simulink model "non_linear_model"  (Simulink 7.3)
settings: Solver=ode45  StartTime=0.0  StopTime=0.01  FixedStep=0.000001  RelTol=1e-1
libraries: simulink x3
settings Model: Creator=alex  LastModifiedBy=alex  BufferReuse=off
settings DataIOCC: SignalLoggingName=sigsOut
settings OptimizationCC: InlineInvariantSignals=on  OptimizeBlockIOStorage=off  BufferReuse=off  ExpressionFolding=off  LocalBlockOutputs=off
settings DebuggingCC: SaveWithParameterizedLinksMsg=none  SignalResolutionControl=TryResolveAllWithWarning  SolverPrmCheckMsg=none  MultiTaskDSMMsg=warning  MultiTaskCondExecSysMsg=none  StrictBusMsg=None
settings HardwareCC: TargetUnknown=on
settings RTWCC: IncludeERTFirstTime=on

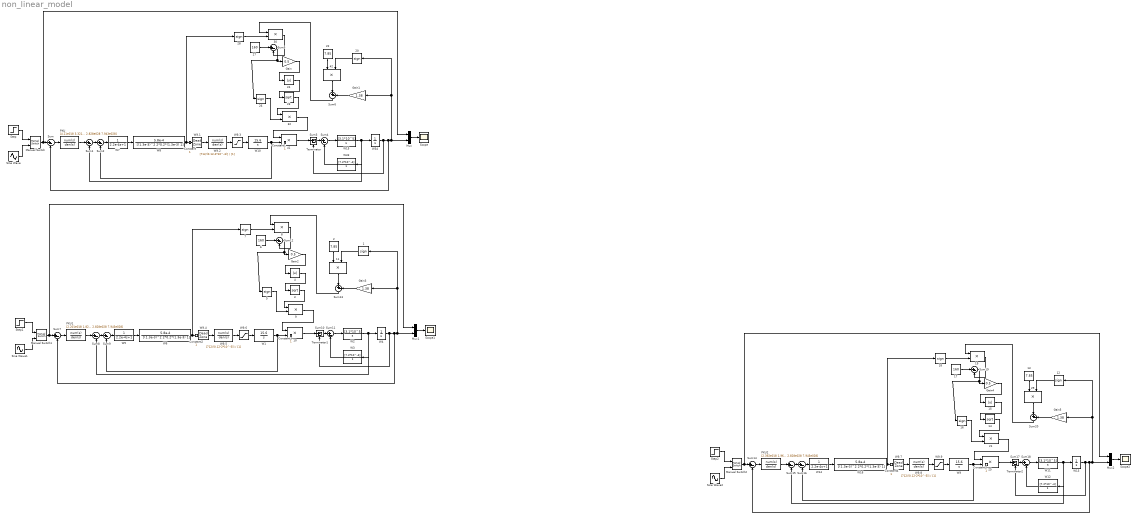
== system non_linear_model ==
  {1,5,7,12,16,18,20,26,28} (9 alike) : Signum
  {8..11,19,21,25,29..30,32,41..42} (12 alike) : Product  OutDataType=sfix(16)  OutScaling=2^0  SaturateOnIntegerOverflow=on  OutDataTypeStr=Inherit: Same as first input
  13 : Constant  Value=7.85  OutDataType=sfix(16)  OutScaling=2^0
  14 : Math  Operator=sqrt  SaturateOnIntegerOverflow=on
  15 : Abs  SaturateOnIntegerOverflow=on
  17 : Constant  Value=160  OutDataType=sfix(16)  OutScaling=2^0
  2 : Constant  Value=7.85  OutDataType=sfix(16)  OutScaling=2^0
  22 : Constant  Value=7.85  OutDataType=sfix(16)  OutScaling=2^0
  23 : Math  Operator=sqrt  SaturateOnIntegerOverflow=on
  24 : Abs  SaturateOnIntegerOverflow=on
  27 : Constant  Value=160  OutDataType=sfix(16)  OutScaling=2^0
  3 : Math  Operator=sqrt  SaturateOnIntegerOverflow=on
  4 : Abs  SaturateOnIntegerOverflow=on
  6 : Constant  Value=160  OutDataType=sfix(16)  OutScaling=2^0
  Constant{,1..5} (6 alike) : Constant  OutDataType=sfix(16)  OutScaling=2^0
  Gain : Gain  Gain=0.5  ParameterDataType=sfix(16)  ParameterScaling=2^0  OutDataType=sfix(16)  OutScaling=2^0  SaturateOnIntegerOverflow=on  OutDataTypeStr=Inherit: Same as input  ParamDataTypeStr=Inherit: Same as input
  Gain1 : Gain  Gain=1.38  ParameterDataType=sfix(16)  ParameterScaling=2^0  OutDataType=sfix(16)  OutScaling=2^0  SaturateOnIntegerOverflow=on  OutDataTypeStr=Inherit: Same as input  ParamDataTypeStr=Inherit: Same as input
  Gain2 : Gain  Gain=0.5  ParameterDataType=sfix(16)  ParameterScaling=2^0  OutDataType=sfix(16)  OutScaling=2^0  SaturateOnIntegerOverflow=on  OutDataTypeStr=Inherit: Same as input  ParamDataTypeStr=Inherit: Same as input
  Gain3 : Gain  Gain=1.38  ParameterDataType=sfix(16)  ParameterScaling=2^0  OutDataType=sfix(16)  OutScaling=2^0  SaturateOnIntegerOverflow=on  OutDataTypeStr=Inherit: Same as input  ParamDataTypeStr=Inherit: Same as input
  Gain4 : Gain  Gain=0.5  ParameterDataType=sfix(16)  ParameterScaling=2^0  OutDataType=sfix(16)  OutScaling=2^0  SaturateOnIntegerOverflow=on  OutDataTypeStr=Inherit: Same as input  ParamDataTypeStr=Inherit: Same as input
  Gain5 : Gain  Gain=1.38  ParameterDataType=sfix(16)  ParameterScaling=2^0  OutDataType=sfix(16)  OutScaling=2^0  SaturateOnIntegerOverflow=on  OutDataTypeStr=Inherit: Same as input  ParamDataTypeStr=Inherit: Same as input
  Manual Switch : simulink/Signal Routing/Manual Switch  SystemSampleTime=-1  sw=0  action=0  varsize=off
  Manual Switch1 : simulink/Signal Routing/Manual Switch  SystemSampleTime=-1  sw=1  action=0  varsize=off
  Manual Switch2 : simulink/Signal Routing/Manual Switch  SystemSampleTime=-1  sw=1  action=0  varsize=off
  Mux : Mux  Inputs=2
  Mux1 : Mux  Inputs=2
  Mux2 : Mux  Inputs=2
  PKU : TransferFcn  Numerator=[4.21e018 3.321e022 3.166e025 2.763e028 1.24e031 1.68e033 5.269e034 + 9.532e032]  Denominator=[1 1.539e006 8.565e011 2.152e017 2.439e022 1.001e027 2.828e028 7.943e028]
  PKU1 : TransferFcn  Numerator=[2.201e018 1.827e022 2.334e025 1.822e028 1.075e031 1.624e033 5.269e034 9.532e032]  Denominator=[1 1.539e006 8.565e011 2.152e017 2.439e022 1.001e027 2.828e028 7.943e028]
  PKU2 : TransferFcn  Numerator=[2.392e018 1.969e022 2.413e025 1.912e028 1.091e031 1.63e033 5.269e034 9.532e032]  Denominator=[1 1.539e006 8.565e011 2.152e017 2.439e022 1.001e027 2.828e028 7.943e028]
  Scope : Scope
      settings: TimeRange=0.003  YMin=0.675  YMax=1
  Scope1 : Scope
      settings: TimeRange=0.003  YMin=0  YMax=1.1
  Scope2 : Scope
      settings: TimeRange=0.003  YMin=0  YMax=1.1  SaveName=ScopeData2
  Sine Wave : Sin  Amplitude=1  Bias=0  Frequency=1200  Phase=0  Samples=10  SampleTime=0  Offset=0
  Sine Wave1 : Sin  Amplitude=1  Bias=0  Frequency=1200  Phase=0  Samples=10  SampleTime=0  Offset=0
  Sine Wave2 : Sin  Amplitude=1  Bias=0  Frequency=1200  Phase=0  Samples=10  SampleTime=0  Offset=0
  Step : Step  Time=0  SampleTime=0
  Step1 : Step  Time=0  SampleTime=0
  Step2 : Step  Time=0  SampleTime=0
  Sum{,1..20} (21 alike) : Sum  Inputs=|+-  OutDataType=sfix(16)  OutScaling=2^0  SaturateOnIntegerOverflow=on
  Terminator : Terminator
  Terminator1 : Terminator
  Terminator2 : Terminator
  W1 : TransferFcn  Numerator=[15.6]  Denominator=[1 0]
  W10 : TransferFcn  Numerator=[15.6]  Denominator=[1 0]
  W11 : TransferFcn  Numerator=[3.1*10^5]  Denominator=[1 0]
  W12 : TransferFcn  Numerator=[7.2*10^-4]  Denominator=[1]
  W13 : TransferFcn  Denominator=[1 0]
  W14 : TransferFcn  Denominator=[2.2e-4 1]
  W15 : TransferFcn  Numerator=[3.1*10^5]  Denominator=[1 0]
  W16 : TransferFcn  Numerator=[5.8e-4]  Denominator=[(1.3e-3)^2 2*0.2*(1.3e-3) 1]
  W2 : TransferFcn  Numerator=[3.1*10^5]  Denominator=[1 0]
  W3 : TransferFcn  Numerator=[7.2*10^-4]  Denominator=[1]
  W33 : TransferFcn  Numerator=[7.2*10^-4]  Denominator=[1]
  W34 : TransferFcn  Denominator=[1 0]
  W4 : TransferFcn  Denominator=[1 0]
  W5 : TransferFcn  Denominator=[2.2e-4 1]
  W6 : TransferFcn  Numerator=[5.8e-4]  Denominator=[(1.3e-3)^2 2*0.2*(1.3e-3) 1]
  W7 : TransferFcn  Denominator=[2.2e-4 1]
  W8 : TransferFcn  Numerator=[5.8e-4]  Denominator=[(1.3e-3)^2 2*0.2*(1.3e-3) 1]
  W9 : TransferFcn  Numerator=[15.6]  Denominator=[1 0]
  W9.1 : DeadZone  LowerValue=-10^-4  UpperValue=10^-4  SaturateOnIntegerOverflow=on
  W9.2 : TransferFcn  Numerator=[712/(0.12-2*10^-3)]  Denominator=[1]
  W9.3 : Saturate  UpperLimit=712  LowerLimit=-712
  W9.4 : DeadZone  LowerValue=-10^-4  UpperValue=10^-4  SaturateOnIntegerOverflow=on
  W9.5 : TransferFcn  Numerator=[712/(0.12-2*10^-3)]  Denominator=[1]
  W9.6 : Saturate  UpperLimit=712  LowerLimit=-712
  W9.7 : DeadZone  LowerValue=-10^-4  UpperValue=10^-4  SaturateOnIntegerOverflow=on
  W9.8 : TransferFcn  Numerator=[712/(0.12-2*10^-3)]  Denominator=[1]
  W9.9 : Saturate  UpperLimit=712  LowerLimit=-712
  wires:
  Sum2/1 -> W7/1
  W7/1 -> W8/1
  Sum3/1 -> Sum4/1
  Sum4/1 -> W15/1
  W15/1 -> Sum1/2, W34/1, W33/1
  Step/1 -> Manual Switch/1
  Sine Wave/1 -> Manual Switch/2
  Mux/1 -> Scope/1
  Manual Switch/1 -> Mux/1, Sum/1
  Sum1/1 -> Sum2/1
  Sum/1 -> PKU/1
  W34/1 -> Sum3/2, Sum/2, Mux/2, Gain1/1, 20/1
  W33/1 -> Sum4/2
  PKU/1 -> Sum1/1
  23/1 -> 32/1
  24/1 -> 23/1
  Gain/1 -> 24/1
  26/1 -> 32/2
  Sum5/1 -> Gain/1, 26/1
  27/1 -> Sum5/1
  30/1 -> Sum5/2
  28/1 -> 30/2
  22/1 -> 42/1
  20/1 -> 42/2
  42/1 -> Sum6/1
  Gain1/1 -> Sum6/2
  Sum6/1 -> 30/1
  32/1 -> 41/1
  W9.2/1 -> W9.3/1
  W8/1 -> W9.1/1, 28/1
  41/1 -> Terminator/1
  W10/1 -> Sum2/2, Sum3/1
  W9.1/1 -> W10/1
  W9.3/1 -> 41/2
  Constant/1 -> W9.2/1
  Sum9/1 -> W5/1
  W5/1 -> W6/1
  Sum10/1 -> Sum11/1
  Sum11/1 -> W2/1
  W2/1 -> Sum8/2, W4/1, W3/1
  Step1/1 -> Manual Switch1/1
  Sine Wave1/1 -> Manual Switch1/2
  Mux1/1 -> Scope1/1
  Manual Switch1/1 -> Mux1/1, Sum7/1
  Sum8/1 -> Sum9/1
  Sum7/1 -> PKU1/1
  W4/1 -> Sum10/2, Sum7/2, Mux1/2, Gain3/1, 1/1
  W3/1 -> Sum11/2
  PKU1/1 -> Sum8/1
  3/1 -> 9/1
  4/1 -> 3/1
  Gain2/1 -> 4/1
  5/1 -> 9/2
  Sum12/1 -> Gain2/1, 5/1
  6/1 -> Sum12/1
  8/1 -> Sum12/2
  7/1 -> 8/2
  2/1 -> 11/1
  1/1 -> 11/2
  11/1 -> Sum13/1
  Gain3/1 -> Sum13/2
  Sum13/1 -> 8/1
  9/1 -> 10/1
  W9.5/1 -> W9.6/1
  W6/1 -> W9.4/1, 7/1
  10/1 -> Terminator1/1
  W1/1 -> Sum9/2, Sum10/1
  W9.4/1 -> W1/1
  W9.6/1 -> 10/2
  Constant2/1 -> W9.5/1
  Sum16/1 -> W14/1
  W14/1 -> W16/1
  Sum17/1 -> Sum18/1
  Sum18/1 -> W11/1
  W11/1 -> Sum15/2, W13/1, W12/1
  Step2/1 -> Manual Switch2/1
  Sine Wave2/1 -> Manual Switch2/2
  Mux2/1 -> Scope2/1
  Manual Switch2/1 -> Mux2/1, Sum14/1
  Sum15/1 -> Sum16/1
  Sum14/1 -> PKU2/1
  W13/1 -> Sum17/2, Sum14/2, Mux2/2, Gain5/1, 12/1
  W12/1 -> Sum18/2
  PKU2/1 -> Sum15/1
  14/1 -> 21/1
  15/1 -> 14/1
  Gain4/1 -> 15/1
  16/1 -> 21/2
  Sum19/1 -> Gain4/1, 16/1
  17/1 -> Sum19/1
  19/1 -> Sum19/2
  18/1 -> 19/2
  13/1 -> 29/1
  12/1 -> 29/2
  29/1 -> Sum20/1
  Gain5/1 -> Sum20/2
  Sum20/1 -> 19/1
  21/1 -> 25/1
  W9.8/1 -> W9.9/1
  W16/1 -> W9.7/1, 18/1
  25/1 -> Terminator2/1
  W9/1 -> Sum16/2, Sum17/1
  W9.7/1 -> W9/1
  W9.9/1 -> 25/2
  Constant4/1 -> W9.8/1
